simulink library "roblocks"  (Simulink 3.00)
values from neighbouring files (symbols this model uses):
  p560 = robot(L, 'Puma 560', 'Unimation', 'params of 8/95')    [puma560.m]
  q = rr.q    [drivebot.m]    (also in fdyn.m = x(1:n); ikine.m = q + dq; inertia.m = q(:)'; maniplty.m = q(:)')
  tau = zeros(n,1)    [fdyn.m]    (also in rne.m = zeros(np,n); rtidemo.m = rne(p560, q, qd, qdd))
undefined symbols (not defined in the file or in its folder): accel, gravity, jacob0
libraries: roblocks x2
settings Model: Creator=pic  LastModifiedBy=pic

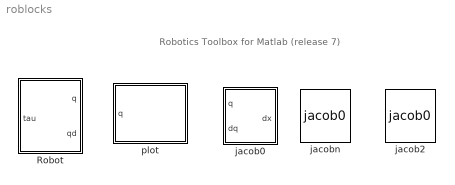
== system roblocks ==
  note: Robotics Toolbox for Matlab (release 7)
  Robot : Subsystem  mask{robot=, q0=}
      mask prompts: robot "Robot object"; q0 "Initial state"
      mask help: Dynamic model of robot
      mask init:
      | n = robot.n;
      mask Help: gravity comes from the robot object
      mask Display:
      | text(0.5, 0.2, robot.name,  'horizontalAlignment', 'center')
      | port_label('input', 1, '\tau')
      | port_label('output', 1, 'q')
      | port_label('output', 2, 'qd')
  jacob0 : Subsystem  mask{robot=}
      mask prompts: robot "Robot object"
      mask help: Robot Jacobian for end-effector coordinates
      mask Display:
      | text(0.4, 0.7, 'J', 'verticalAlignment', 'top', 'horizontalAlignment', 'left')
      | text(0.4, 0.7, '0', 'verticalAlignment', 'bottom', 'horizontalAlignment', 'right')
      | text(0.5, 0.2, robot.name,  'horizontalAlignment', 'center')
  jacob2 : roblocks/jacob0
  jacobn : roblocks/jacob0
  plot : Subsystem  mask{robot=p560}
      mask prompts: robot "Name of robot"
      mask init:
      | plot(robot,zeros(robot.n,1))
      mask Help: This block graphically displays the named robot
      mask Display: text(0.5, 0.5,  robot.name, 'horizontalAlignment', 'center')

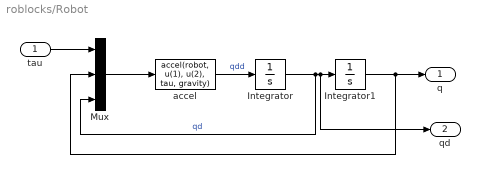
== system roblocks/Robot ==
  tau : Inport  Port=1  PortWidth=-1  SampleTime=-1  DataType=auto
      settings: SignalType=auto
  Integrator : Integrator  ExternalReset=none  InitialConditionSource=internal  InitialCondition=0  LimitOutput=off  UpperSaturationLimit=inf  LowerSaturationLimit=-inf  ShowSaturationPort=off  ShowStatePort=off  AbsoluteTolerance=auto
  Integrator1 : Integrator  ExternalReset=none  InitialConditionSource=internal  InitialCondition=0  LimitOutput=off  UpperSaturationLimit=inf  LowerSaturationLimit=-inf  ShowSaturationPort=off  ShowStatePort=off  AbsoluteTolerance=auto
  Mux : Mux  Inputs=3
  accel : Fcn  Expr=accel(robot, u(1), u(2), tau, gravity)
  q : Outport  Port=1
  qd : Outport  Port=2
  wires:
  Mux/1 -> accel/1
  tau/1 -> Mux/1
  accel/1 -> Integrator/1  "qdd"
  Integrator1/1 -> q/1, Mux/2
  Integrator/1 -> Integrator1/1, qd/1, Mux/3  "qd"

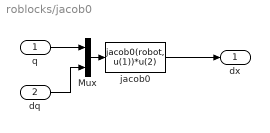
== system roblocks/jacob0 ==
  q : Inport  Port=1  PortWidth=-1  SampleTime=-1  DataType=auto
      settings: SignalType=auto
  dq : Inport  Port=2  PortWidth=-1  SampleTime=-1  DataType=auto
      settings: SignalType=auto
  Mux : Mux  Inputs=2
  jacob0 : Fcn  Expr=jacob0(robot, u(1))*u(2)
  dx : Outport  Port=1
  wires:
  jacob0/1 -> dx/1
  Mux/1 -> jacob0/1
  q/1 -> Mux/1
  dq/1 -> Mux/2

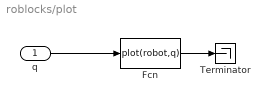
== system roblocks/plot ==
  q : Inport  Port=1  PortWidth=-1  SampleTime=-1  DataType=auto
      settings: SignalType=auto
  Fcn : Fcn  Expr=plot(robot,q)
  Terminator : Terminator
  wires:
  q/1 -> Fcn/1
  Fcn/1 -> Terminator/1
